simulink model "sim_partie_vitesse"  (R2020a)
settings: Solver=VariableStepAuto  StartTime=0.0  StopTime=20  RelTol=1e-3
settings Model: Creator=kttran  LastModifiedBy=kttran

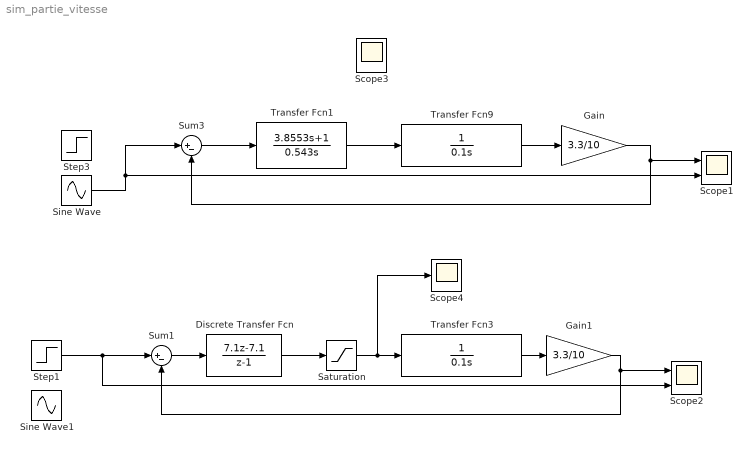
== system sim_partie_vitesse ==
  Discrete Transfer Fcn : DiscreteTransferFcn  Numerator=[7.1 -7.1]  Denominator=[1 -1]
  Gain : Gain  Gain=3.3/10
  Gain1 : Gain  Gain=3.3/10
  Saturation : Saturate  UpperLimit=3.3  LowerLimit=0
  Scope1 : Scope  NumInputPorts=2
  Scope2 : Scope  NumInputPorts=2
  Scope3 : Scope  NumInputPorts=3
  Scope4 : Scope
  Sine Wave : Sin  SampleTime=0
  Sine Wave1 : Sin  SampleTime=0
  Step1 : Step  Time=0.1  SampleTime=0
  Step3 : Step  Time=5e-3  Before=-0.1  After=0.2  SampleTime=0
  Sum1 : Sum  Inputs=|+-
  Sum3 : Sum  Inputs=|+-
  Transfer Fcn1 : TransferFcn  Numerator=[3.8553 1]  Denominator=[0.543 0]
  Transfer Fcn3 : TransferFcn  Denominator=[0.1 0]
  Transfer Fcn9 : TransferFcn  Denominator=[0.1 0]
  wires:
  Sine Wave/1 -> Sum3/1, Scope1/2
  Gain/1 -> Sum3/2, Scope1/1
  Transfer Fcn9/1 -> Gain/1
  Sum1/1 -> Discrete Transfer Fcn/1
  Gain1/1 -> Sum1/2, Scope2/1
  Transfer Fcn3/1 -> Gain1/1
  Discrete Transfer Fcn/1 -> Saturation/1
  Saturation/1 -> Scope4/1, Transfer Fcn3/1
  Step1/1 -> Scope2/2, Sum1/1
  Sum3/1 -> Transfer Fcn1/1
  Transfer Fcn1/1 -> Transfer Fcn9/1
